simulink model "FullWaveRectifier"  (R2018a)
settings: Solver=ode45  StartTime=0.0  StopTime=1.0  RelTol=1e-3
libraries: powerlib x12
settings Model: Creator=chron  LastModifiedBy=chron

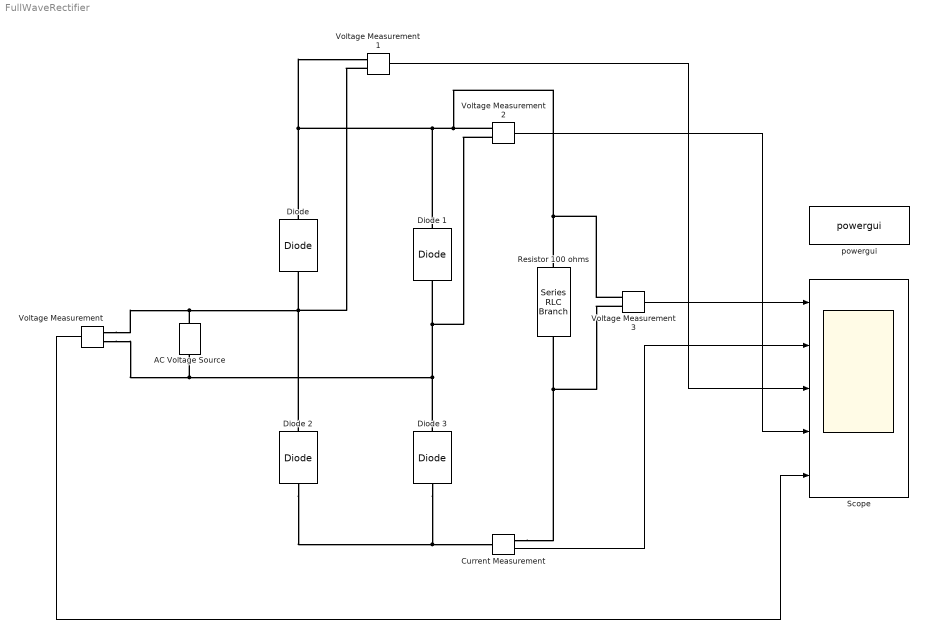
== system FullWaveRectifier ==
  "AC Voltage Source " : powerlib/Electrical Sources/AC Voltage Source  Amplitude=100  Phase=0  Frequency=60  SampleTime=0  Measurements=None  BusType=swing  Pref=10e3  Qref=0  Qmin=-inf  Qmax=+inf
  "Current Measurement " : powerlib/Measurements/Current Measurement  PhasorSimulation=off  OutputType=Complex  PSBequivalent=0
  Diode {,1..3} (4 alike) : powerlib/Power Electronics/Diode  Ron=0.001  Lon=0  Vf=0.8  IC=0  UseSnubber=0  Rs=500  Cs=250e-9  Measurements=off
  Resistor 100 ohms : powerlib/Elements/Series RLC Branch  LConnTagsString=__new0  RConnTagsString=__new0  BranchType=RLC  Resistance=100  Inductance=1e-3  SetiL0=off  InitialCurrent=0  Capacitance=1e-6  Setx0=off  InitialVoltage=0  Measurements=None
  "Scope " : Scope  NumInputPorts=5
  "Voltage Measurement1 " : powerlib/Measurements/Voltage Measurement  PhasorSimulation=off  OutputType=Complex  PSBequivalent=0
  "Voltage Measurement2 " : powerlib/Measurements/Voltage Measurement  PhasorSimulation=off  OutputType=Complex  PSBequivalent=0
  Voltage Measurement : powerlib/Measurements/Voltage Measurement  PhasorSimulation=off  OutputType=Complex  PSBequivalent=0
  "Voltage Measurement3 " : powerlib/Measurements/Voltage Measurement  PhasorSimulation=off  OutputType=Complex  PSBequivalent=0
  "powergui " : powerlib/powergui  Priority=1  SimulationMode=Continuous  SampleTime=50e-6  frequency=60  Iterations=50  frequencyindice=60  Pbase=100e6  ErrMax=1e-4  UnitsV=kV  UnitsW=MW  buscounter=0  FunctionMessages=off  echomessages=off  EnableUseOfTLC=off  CurrentSourceSwitches=off  DisableSnubberDevices=off  DisableRonSwitches=off  DisableVfSwitches=off  DisplayEquations=off  SolverType=Tustin/Backward Euler (TBE)  Interpol=off  ExternalGateDelay=off  methode=off  Ts=100  x0status=blocks  SPID=on  SwTol=0  HookPort=off  RestoreLinks=warning  ResistiveCurrentMeasurement=off  Frange=[0:2:500]  Ylog=off  Xlog=on  ShowGrid=off  save=off  variable=ZData  structure=0  ZoomFFT=off  StartTime=0.0  cycles=1  DisplayStyle=1  fundamental=60  FreqAxis=off  MaxFrequency=1000  frequencyindicesteady=1  RmsSteady=1  display=off
  wires:
  Voltage Measurement/1 -> "Scope "/5
  "Voltage Measurement1 "/1 -> "Scope "/3
  "Voltage Measurement3 "/1 -> "Scope "/1
  "Voltage Measurement2 "/1 -> "Scope "/4
  "Current Measurement "/1 -> "Scope "/2
  connections:
  Voltage Measurement/LConn1 -- "AC Voltage Source "/RConn1 -- Diode 2/LConn1 -- "Voltage Measurement1 "/LConn2 -- "Diode "/RConn1
  "Diode "/LConn1 -- Diode 1/LConn1 -- "Voltage Measurement3 "/LConn2 -- Resistor 100 ohms/LConn1 -- "Voltage Measurement2 "/LConn2 -- "Voltage Measurement1 "/LConn1
  "Current Measurement "/RConn1 -- "Voltage Measurement3 "/LConn1 -- Resistor 100 ohms/RConn1
  Voltage Measurement/LConn2 -- Diode 3/LConn1 -- Diode 1/RConn1 -- "Voltage Measurement2 "/LConn1 -- "AC Voltage Source "/LConn1
  Diode 3/RConn1 -- Diode 2/RConn1 -- "Current Measurement "/LConn1
